simulink model "quadcopter_simu"  (R2024b)
settings: Solver=VariableStepAuto  StartTime=0.0  StopTime=10.0  RelTol=1e-3
values from neighbouring files (symbols this model uses):
  A = [ ... (first row only)    [quadcopter.m]
  B = [1, 0]    [quadcopter.m]
  C = [0, 1]    [quadcopter.m]
  K = [1, 0]    [quadcopter.m]
  L = [1; 0]    [quadcopter.m]
  N = [1, 1]    [quadcopter.m]
  r = 0    [quadcopter.m]
settings Model: Creator=jonas  LastModifiedBy=jonas

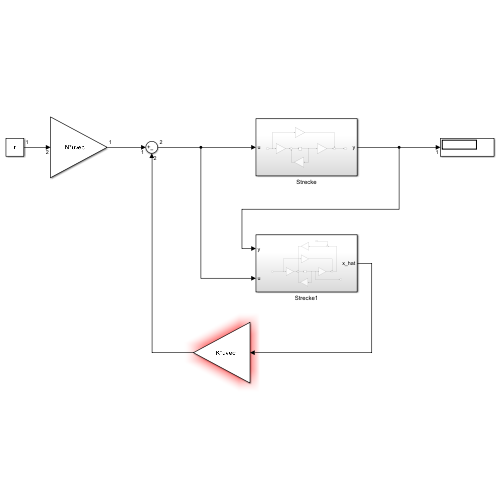
[thumbnail: Simulink's stored preview of the top-level diagram]
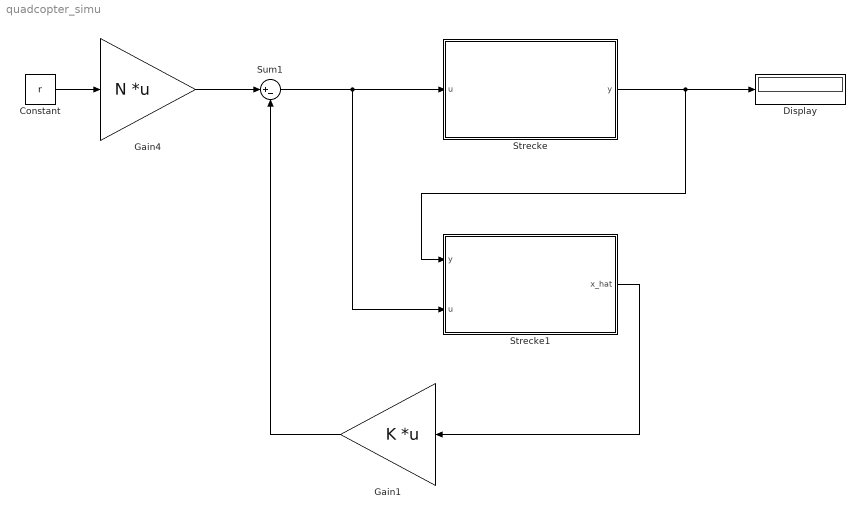
== system quadcopter_simu ==
  Constant : Constant  Value=r
  Display : Display
  Gain1 : Gain  Description=B  Gain=K  Multiplication=Matrix(K*u) (u vector)
  Gain4 : Gain  Description=B  Gain=N  Multiplication=Matrix(K*u) (u vector)
  Strecke : Subsystem
  Strecke1 : Subsystem
  Sum1 : Sum  Inputs=|+-
  wires:
  Constant/1 -> Gain4/1
  Gain4/1 -> Sum1/1
  Sum1/1 -> Strecke1/2(u), Strecke/1(u)
  Strecke/1(y) -> Strecke1/1(y), Display/1
  Strecke1/1(x_hat) -> Gain1/1
  Gain1/1 -> Sum1/2

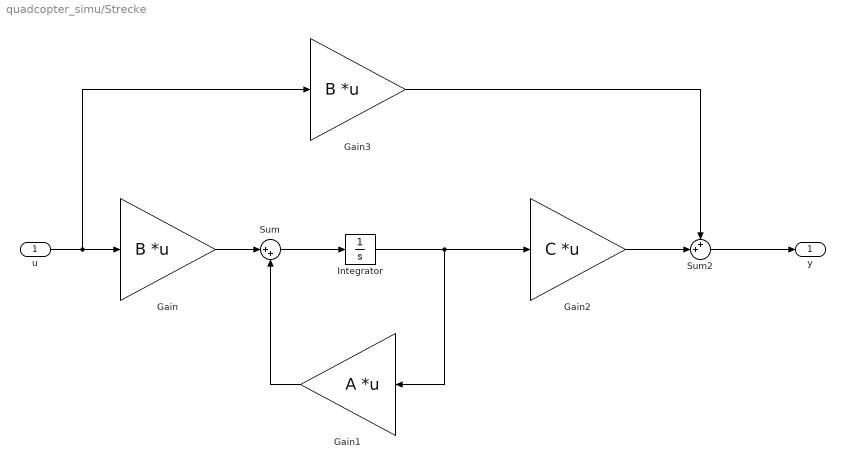
== system quadcopter_simu/Strecke ==
  u : Inport
  Gain : Gain  Description=B  Gain=B  Multiplication=Matrix(K*u) (u vector)
  Gain1 : Gain  Description=B  Gain=A  Multiplication=Matrix(K*u) (u vector)
  Gain2 : Gain  Description=B  Gain=C  Multiplication=Matrix(K*u) (u vector)
  Gain3 : Gain  Description=B  Gain=B  Multiplication=Matrix(K*u) (u vector)
  Integrator : Integrator
  Sum : Sum  Inputs=|++
  Sum2 : Sum  Inputs=++|
  y : Outport
  wires:
  Gain3/1 -> Sum2/1
  Gain2/1 -> Sum2/2
  Integrator/1 -> Gain2/1, Gain1/1
  u/1 -> Gain3/1, Gain/1
  Gain/1 -> Sum/1
  Sum/1 -> Integrator/1
  Gain1/1 -> Sum/2
  Sum2/1 -> y/1

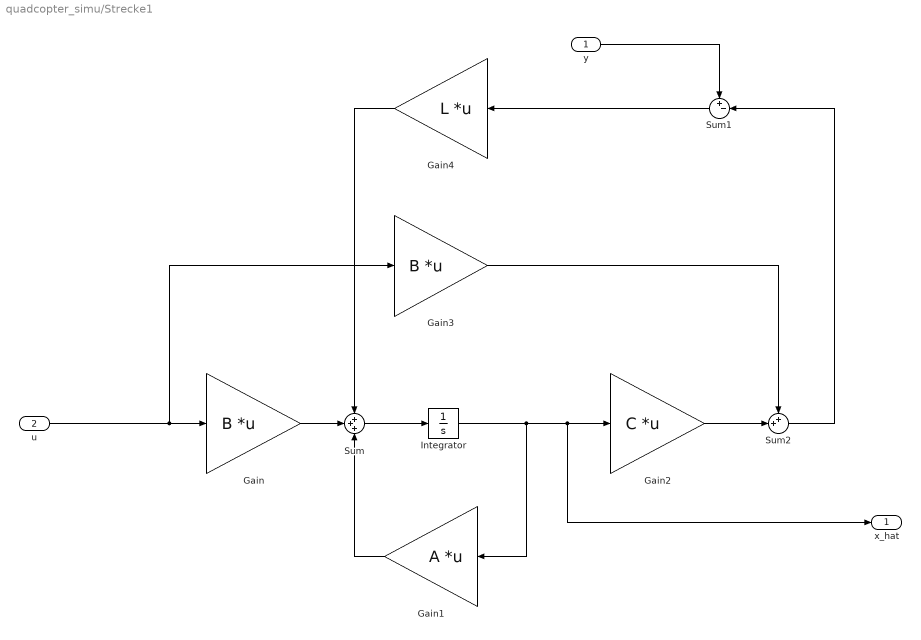
== system quadcopter_simu/Strecke1 ==
  y : Inport
  u : Inport  Port=2
  Gain : Gain  Description=B  Gain=B  Multiplication=Matrix(K*u) (u vector)
  Gain1 : Gain  Description=B  Gain=A  Multiplication=Matrix(K*u) (u vector)
  Gain2 : Gain  Description=B  Gain=C  Multiplication=Matrix(K*u) (u vector)
  Gain3 : Gain  Description=B  Gain=B  Multiplication=Matrix(K*u) (u vector)
  Gain4 : Gain  Description=B  Gain=L  Multiplication=Matrix(K*u) (u vector)
  Integrator : Integrator
  Sum : Sum  Inputs=+++
  Sum1 : Sum  Inputs=+-|
  Sum2 : Sum  Inputs=++|
  x_hat : Outport
  wires:
  Gain3/1 -> Sum2/1
  Gain2/1 -> Sum2/2
  Integrator/1 -> x_hat/1, Gain2/1, Gain1/1
  u/1 -> Gain3/1, Gain/1
  Sum/1 -> Integrator/1
  Sum2/1 -> Sum1/2
  Gain1/1 -> Sum/3
  Gain/1 -> Sum/2
  y/1 -> Sum1/1
  Sum1/1 -> Gain4/1
  Gain4/1 -> Sum/1
